simulink model "three_phase_pll_real"  (R2022a)
settings: Solver=VariableStepAuto  StartTime=0.0  StopTime=5  RelTol=1e-3
values from neighbouring files (symbols this model uses):
  Ki_pll = (Wn^2) / A    (= 394784.176044)    [q1.m]    (also in q4.m = 1579136.70417)
  Kp_pll = 2*DF / sqrt(A/Ki_pll)    [q1.m]    (also in q4.m = 2*DF / sqrt(1/Ki_pll))
  Tcs = 100*Ts    (= 0.0001)    [q1.m]    (also in q4.m)
libraries: simulink_extras x3, spsabctodq0Lib x1
settings Model: Creator=fiendchain  LastModifiedBy=acidi

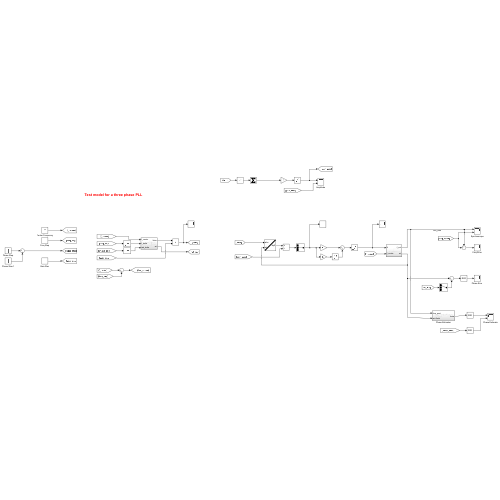
[thumbnail: Simulink's stored preview of the top-level diagram]
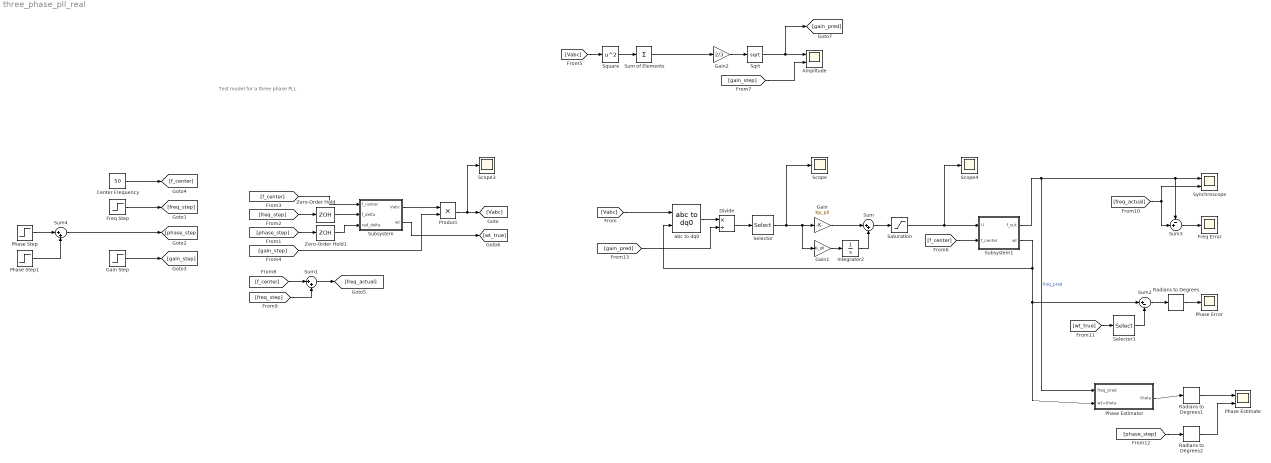
== system three_phase_pll_real ==
  note: Test model for a three phase PLL
  Amplitude : Scope  NumInputPorts=2
  Center Frequency : Constant  Value=50
  Divide : Product  Inputs=*/
  Freq Error : Scope
  Freq Step : Step  After=-2  SampleTime=0
  Gain : Gain  Gain=Kp_pll
  Gain Step : Step  Time=3  Before=400*sqrt(2)  After=400*sqrt(2)*0.2  SampleTime=1/10000
  Gain1 : Gain  Gain=Ki_pll
  Gain2 : Gain  Gain=2/3
  Integrator2 : Integrator  LimitOutput=on  UpperSaturationLimit=2*pi*10  LowerSaturationLimit=-2*pi*10
  Phase Error : Scope
  Phase Estimate : Scope  NumInputPorts=2
  Phase Estimator : Subsystem
  Phase Step : Step  Time=2  After=15 * pi/180  SampleTime=0
  Phase Step1 : Step  Time=4  After=-25 * pi/180  SampleTime=0
  Product : Product
  Radians to Degrees : simulink_extras/Transformations/Radians to Degrees
  Radians to Degrees1 : simulink_extras/Transformations/Radians to Degrees
  Radians to Degrees2 : simulink_extras/Transformations/Radians to Degrees
  Saturation : Saturate  UpperLimit=2*pi*5  LowerLimit=-2*pi*5
  Scope : Scope
  Scope3 : Scope
  Scope4 : Scope
  Selector : Selector  InputPortWidth=3  IndexOptions=Index vector (dialog)  Indices=[2]  OutputSizes=1
  Selector1 : Selector  InputPortWidth=3  IndexOptions=Index vector (dialog)  Indices=[1]  OutputSizes=1
  Sqrt : Sqrt
  Square : Math  Operator=square
  Subsystem : Subsystem
  Subsystem1 : Subsystem
  Sum : Sum  Inputs=|++
  Sum of Elements : Sum  Inputs=+
  Sum1 : Sum  Inputs=|++
  Sum2 : Sum  Inputs=|+-
  Sum3 : Sum  Inputs=-+|
  Sum4 : Sum  Inputs=|++
  Synchroscope : Scope  NumInputPorts=2
  Zero-Order Hold : ZeroOrderHold  SampleTime=Tcs
  Zero-Order Hold1 : ZeroOrderHold  SampleTime=Tcs
  abc to dq0 : spsabctodq0Lib/abc to dq0  Alignment=Aligned with phase A axis
  wires:
  Divide/1 -> Selector/1
  Gain/1 -> Sum/1
  Gain1/1 -> Integrator2/1
  Integrator2/1 -> Sum/2
  Selector/1 -> Scope/1, Gain1/1, Gain/1
  Zero-Order Hold/1 -> Subsystem/2(f_delta)
  Product/1 -> Scope3/1, [Vabc]
  Subsystem/1(Vabc) -> Product/1
  Zero-Order Hold1/1 -> Subsystem/3(rad_delta)
  Subsystem1/2(wt) -> Phase Estimator/2(wt+theta), Sum2/1, abc to dq0/2
  Subsystem1/1(f_out) -> Phase Estimator/1(freq_pred), Synchroscope/1, Sum3/1  "freq_pred"
  [f_center] -> Subsystem1/2(f_center)
  Sum/1 -> Saturation/1
  Saturation/1 -> Scope4/1, Subsystem1/1(U)
  Square/1 -> Sum of Elements/1
  Gain2/1 -> Sqrt/1
  Sum of Elements/1 -> Gain2/1
  [Vabc] -> abc to dq0/1
  Center Frequency/1 -> [f_center]
  Freq Step/1 -> [freq_step]
  Gain Step/1 -> [gain_step]
  Sum4/1 -> [phase_step]
  [phase_step] -> Zero-Order Hold1/1
  [freq_step] -> Zero-Order Hold/1
  [f_center] -> Subsystem/1(f_center)
  [gain_step] -> Product/2
  [Vabc] -> Square/1
  [gain_step] -> Amplitude/2
  Sum1/1 -> [freq_actual]
  [freq_step] -> Sum1/2
  [f_center] -> Sum1/1
  [freq_actual] -> Sum3/2, Synchroscope/2
  Subsystem/2(wt) -> [wt_true]
  [wt_true] -> Selector1/1
  Sum2/1 -> Radians to Degrees/1
  Selector1/1 -> Sum2/2
  Radians to Degrees/1 -> Phase Error/1
  Sum3/1 -> Freq Error/1
  Sqrt/1 -> [gain_pred], Amplitude/1
  [phase_step] -> Radians to Degrees2/1
  Radians to Degrees2/1 -> Phase Estimate/2
  Phase Estimator/1(theta) -> Radians to Degrees1/1
  Radians to Degrees1/1 -> Phase Estimate/1
  Phase Step/1 -> Sum4/1
  Phase Step1/1 -> Sum4/2
  abc to dq0/1 -> Divide/1
  [gain_pred] -> Divide/2

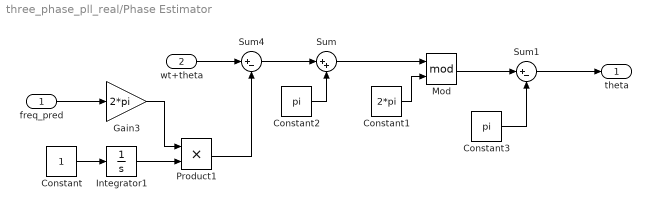
== system three_phase_pll_real/Phase Estimator ==
  freq_pred : Inport
  wt+theta : Inport  Port=2
  Constant : Constant
  Constant1 : Constant  Value=2*pi
  Constant2 : Constant  Value=pi
  Constant3 : Constant  Value=pi
  Gain3 : Gain  Gain=2*pi
  Integrator1 : Integrator
  Mod : Math  Operator=mod
  Product1 : Product
  Sum : Sum  Inputs=|++
  Sum1 : Sum  Inputs=|+-
  Sum4 : Sum  Inputs=|+-
  theta : Outport
  wires:
  Product1/1 -> Sum4/2
  wt+theta/1 -> Sum4/1
  Gain3/1 -> Product1/1
  Sum/1 -> Mod/1
  Constant/1 -> Integrator1/1
  freq_pred/1 -> Gain3/1
  Constant1/1 -> Mod/2
  Integrator1/1 -> Product1/2
  Sum1/1 -> theta/1
  Sum4/1 -> Sum/1
  Constant2/1 -> Sum/2
  Mod/1 -> Sum1/1
  Constant3/1 -> Sum1/2

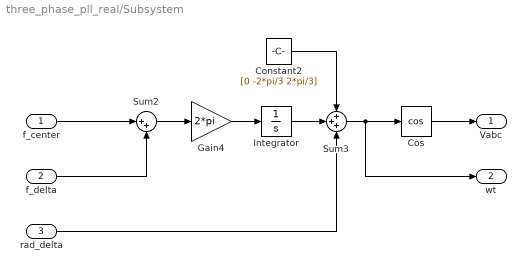
== system three_phase_pll_real/Subsystem ==
  f_center : Inport
  f_delta : Inport  Port=2
  rad_delta : Inport  Port=3
  Constant2 : Constant  Value=[0 -2*pi/3 2*pi/3]
  Cos : Trigonometry  Operator=cos
  Gain4 : Gain  Gain=2*pi
  Integrator : Integrator
  Sum2 : Sum  Inputs=|++
  Sum3 : Sum  Inputs=+++
  Vabc : Outport
  wt : Outport  Port=2
  wires:
  Sum3/1 -> wt/1, Cos/1
  Sum2/1 -> Gain4/1
  Gain4/1 -> Integrator/1
  Cos/1 -> Vabc/1
  f_delta/1 -> Sum2/2
  f_center/1 -> Sum2/1
  rad_delta/1 -> Sum3/3
  Integrator/1 -> Sum3/2
  Constant2/1 -> Sum3/1

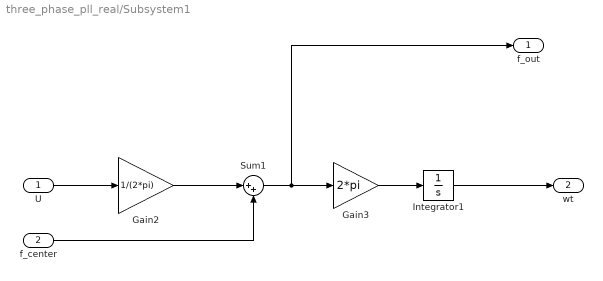
== system three_phase_pll_real/Subsystem1 ==
  U : Inport
  f_center : Inport  Port=2
  Gain2 : Gain  Gain=1/(2*pi)
  Gain3 : Gain  Gain=2*pi
  Integrator1 : Integrator
  Sum1 : Sum  Inputs=|++
  f_out : Outport
  wt : Outport  Port=2
  wires:
  Gain3/1 -> Integrator1/1
  f_center/1 -> Sum1/2
  Gain2/1 -> Sum1/1
  Integrator1/1 -> wt/1
  U/1 -> Gain2/1
  Sum1/1 -> f_out/1, Gain3/1
